simulink library "Game_Development_Library"  (R2024a)
settings: Solver=VariableStepAuto  StartTime=0.0  StopTime=10.0  RelTol=1e-3
libraries: simulink x6
settings Model: Creator=alfa  LastModifiedBy=alfa

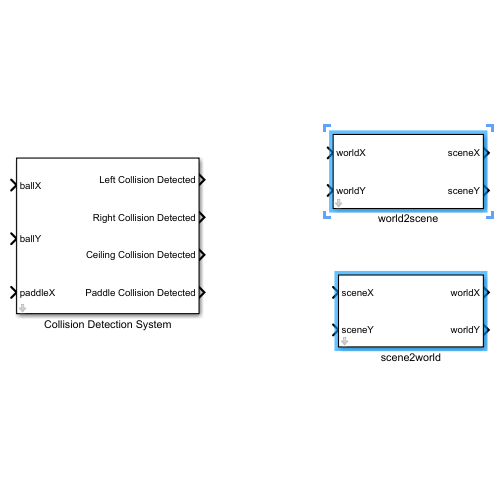
[thumbnail: Simulink's stored preview of the top-level diagram]
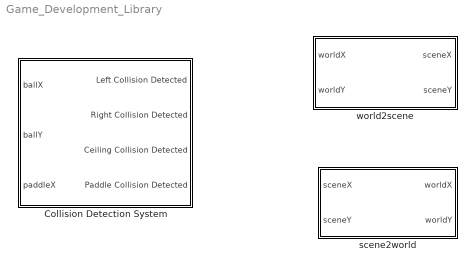
== system Game_Development_Library ==
  Collision Detection System : Subsystem  mask(X- and Y-coordinates of walls and ceilings, width of walls, radius of ball){X_left=-3, X_right=3, w=0.3, Y_ceiling=6, r=0}
      mask prompts: X_left "X-coordinate of left wall"; X_right "X-coordinate of right wall"; w "Width of wall"; Y_ceiling "Y-coordinate of ceiling"; r "Radius of ball"
  scene2world : Subsystem  mask{w=0, h=0}
      mask prompts: w "Width"; h "Height"
  world2scene : Subsystem  mask(world2scene){w=2000, h=250}
      mask prompts: w "Width"; h "Height"

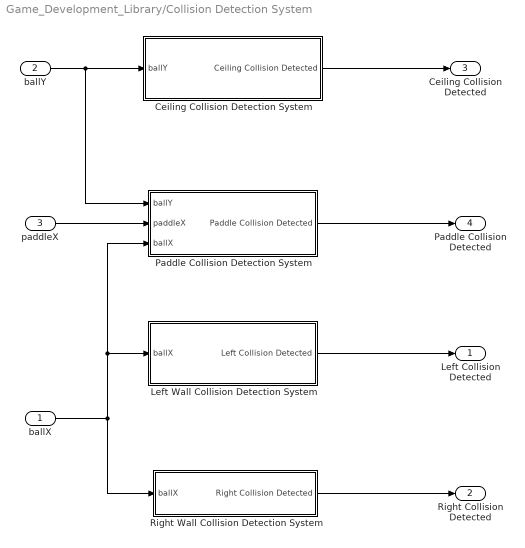
== system Game_Development_Library/Collision Detection System ==
  ballX : Inport
  ballY : Inport  Port=2
  paddleX : Inport  Port=3
  Ceiling Collision Detection System : Subsystem  mask(Y-coordinate used to draw rectangle forming the ceiling, ball radius){Y_ceiling=6, r=0}
      mask prompts: Y_ceiling "Y-coordinate of ceiling"; r "Radius of ball"
  Left Wall Collision Detection System : Subsystem  mask(X-coordinate used to draw rectangle forming the left wall and its' width, ball radius){w=0.3, X_left=-3, r=0}
      mask prompts: w "Width of the wall"; X_left "X-coordinate of left wall"; r "Radius of ball"
  Paddle Collision Detection System : Subsystem  mask{w_paddle=0, h_paddle=0, paddleY=0, r=0}
      mask prompts: w_paddle "Width of paddle"; h_paddle "Height of paddle"; paddleY "Y-coordinate of paddle"; r "Radius of ball"
  Right Wall Collision Detection System : Subsystem  mask(X-coordinate used to draw rectangle forming the right wall, ball radius){X_right=3, r=0}
      mask prompts: X_right "X-coordinate of right wall"; r "Radius of ball"
  Left Collision Detected : Outport
  Right Collision Detected : Outport  Port=2
  Ceiling Collision Detected : Outport  Port=3
  Paddle Collision Detected : Outport  Port=4
  wires:
  Paddle Collision Detection System/1(Paddle Collision Detected) -> Paddle Collision Detected/1
  paddleX/1 -> Paddle Collision Detection System/2(paddleX)
  ballY/1 -> Ceiling Collision Detection System/1(ballY), Paddle Collision Detection System/1(ballY)
  Ceiling Collision Detection System/1(Ceiling Collision Detected) -> Ceiling Collision Detected/1
  Left Wall Collision Detection System/1(Left Collision Detected) -> Left Collision Detected/1
  Right Wall Collision Detection System/1(Right Collision Detected) -> Right Collision Detected/1
  ballX/1 -> Left Wall Collision Detection System/1(ballX), Paddle Collision Detection System/3(ballX), Right Wall Collision Detection System/1(ballX)

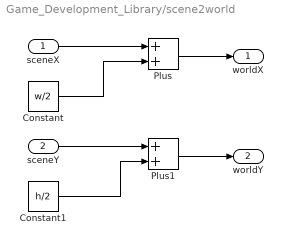
== system Game_Development_Library/scene2world ==
  sceneX : Inport
  "sceneY " : Inport  Port=2
  Constant : Constant  Value=w/2
  Constant1 : Constant  Value=h/2
  Plus : Sum
  Plus1 : Sum
  worldX : Outport
  worldY : Outport  Port=2
  wires:
  Plus1/1 -> worldY/1
  Constant1/1 -> Plus1/2
  Constant/1 -> Plus/2
  Plus/1 -> worldX/1
  sceneX/1 -> Plus/1
  "sceneY "/1 -> Plus1/1

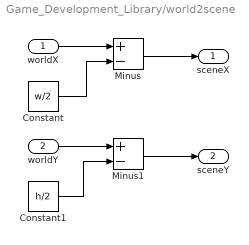
== system Game_Development_Library/world2scene ==
  worldX : Inport
  worldY : Inport  Port=2
  Constant : Constant  Value=w/2
  Constant1 : Constant  Value=h/2
  Minus : Sum  Inputs=+-
  Minus1 : Sum  Inputs=+-
  sceneX : Outport
  sceneY : Outport  Port=2
  wires:
  Minus1/1 -> sceneY/1
  Constant1/1 -> Minus1/2
  worldY/1 -> Minus1/1
  Constant/1 -> Minus/2
  Minus/1 -> sceneX/1
  worldX/1 -> Minus/1

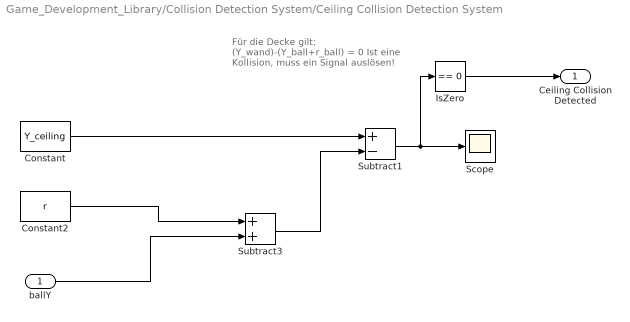
== system Game_Development_Library/Collision Detection System/Ceiling Collision Detection System ==
  note: Für die Decke gilt:
      | (Y_wand)-(Y_ball+r_ball) = 0
      | Ist eine Kollision, muss ein Signal auslösen!
  ballY : Inport
  Constant : Constant  Value=Y_ceiling
  Constant2 : Constant  Value=r
  IsZero : simulink/Logic and Bit Operations/Compare To Zero  relop===  OutDataTypeStr=boolean
      settings: LibrarySourceBlock=|
      | simulink/Quick Insert/Logic and Bit
      | Operations/IsZero
  Scope : Scope
  Subtract1 : Sum  Inputs=+-
  Subtract3 : Sum
  Ceiling Collision Detected : Outport
  wires:
  Constant/1 -> Subtract1/1
  Subtract1/1 -> Scope/1, IsZero/1
  IsZero/1 -> Ceiling Collision Detected/1
  Subtract3/1 -> Subtract1/2
  Constant2/1 -> Subtract3/1
  ballY/1 -> Subtract3/2

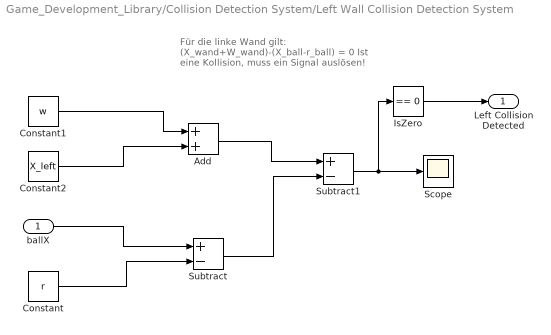
== system Game_Development_Library/Collision Detection System/Left Wall Collision Detection System ==
  note: Für die linke Wand gilt:
      | (X_wand+W_wand)-(X_ball-r_ball) = 0
      | Ist eine Kollision, muss ein Signal auslösen!
  ballX : Inport
  Add : Sum
  Constant : Constant  Value=r
  Constant1 : Constant  Value=w
  Constant2 : Constant  Value=X_left
  IsZero : simulink/Logic and Bit Operations/Compare To Zero  relop===  OutDataTypeStr=boolean
      settings: LibrarySourceBlock=|
      | simulink/Quick Insert/Logic and Bit
      | Operations/IsZero
  Scope : Scope
  Subtract : Sum  Inputs=+-
  Subtract1 : Sum  Inputs=+-
  Left Collision Detected : Outport
  wires:
  Subtract1/1 -> Scope/1, IsZero/1
  ballX/1 -> Subtract/1
  Constant1/1 -> Add/1
  Add/1 -> Subtract1/1
  Constant2/1 -> Add/2
  Subtract/1 -> Subtract1/2
  Constant/1 -> Subtract/2
  IsZero/1 -> Left Collision Detected/1

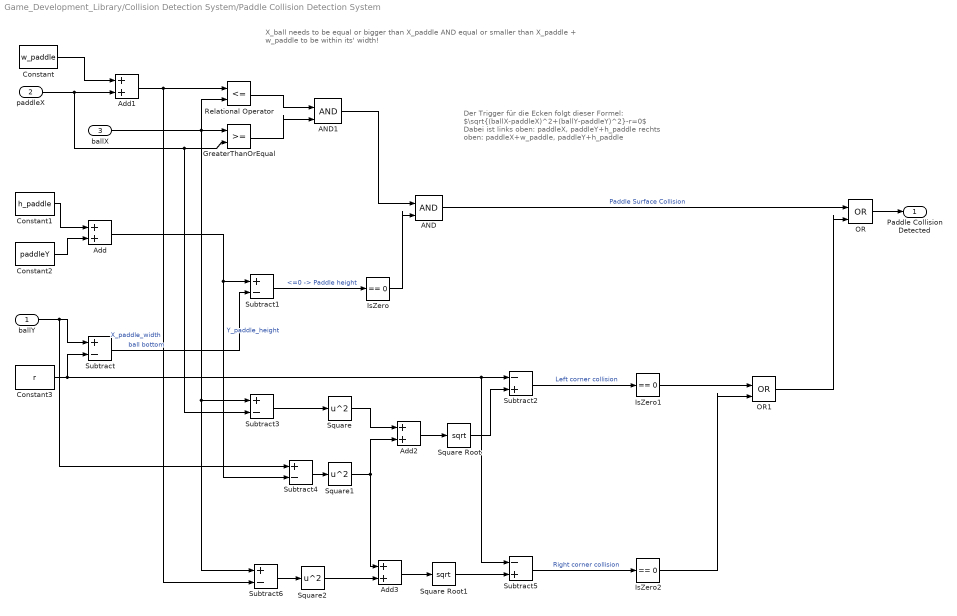
== system Game_Development_Library/Collision Detection System/Paddle Collision Detection System ==
  note: X_ball needs to be equal or bigger than X_paddle AND equal or smaller than X_paddle + w_paddle to be within its' width!
  note: Der Trigger für die Ecken folgt dieser Formel:
      | $\sqrt{(ballX-paddleX)^2+(ballY-paddleY)^2}-r=0$
      |
      | Dabei ist links oben: paddleX, paddleY+h_paddle
      | rechts oben: paddleX+w_paddle, paddleY+h_paddle
  ballY : Inport
  paddleX : Inport  Port=2
  ballX : Inport  Port=3
  AND : Logic  IconShape=distinctive  AllPortsSameDT=off  OutDataTypeStr=boolean
  AND1 : Logic  IconShape=distinctive  AllPortsSameDT=off  OutDataTypeStr=boolean
  Add{,1..3} (4 alike) : Sum
  Constant : Constant  Value=w_paddle
  Constant1 : Constant  Value=h_paddle
  Constant2 : Constant  Value=paddleY
  Constant3 : Constant  Value=r
  GreaterThanOrEqual : RelationalOperator  OutDataTypeStr=boolean  RndMeth=Simplest  InputSameDT=off
  IsZero : simulink/Logic and Bit Operations/Compare To Zero  relop===  OutDataTypeStr=boolean
      settings: LibrarySourceBlock=|
      | simulink/Quick Insert/Logic and Bit
      | Operations/IsZero
  IsZero1 : simulink/Logic and Bit Operations/Compare To Zero  relop===  OutDataTypeStr=boolean
      settings: LibrarySourceBlock=|
      | simulink/Quick Insert/Logic and Bit
      | Operations/IsZero
  IsZero2 : simulink/Logic and Bit Operations/Compare To Zero  relop===  OutDataTypeStr=boolean
      settings: LibrarySourceBlock=|
      | simulink/Quick Insert/Logic and Bit
      | Operations/IsZero
  OR : Logic  Operator=OR  IconShape=distinctive  AllPortsSameDT=off  OutDataTypeStr=boolean
  OR1 : Logic  Operator=OR  IconShape=distinctive  AllPortsSameDT=off  OutDataTypeStr=boolean
  Relational Operator : RelationalOperator  Operator=<=  OutDataTypeStr=boolean  RndMeth=Simplest  InputSameDT=off
  Square : Math  Operator=square
  Square Root : Sqrt
  Square Root1 : Sqrt
  Square1 : Math  Operator=square
  Square2 : Math  Operator=square
  Subtract{,1,3..4,6} (5 alike) : Sum  Inputs=+-
  Subtract2 : Sum  Inputs=-+
  Subtract5 : Sum  Inputs=-+
  Paddle Collision Detected : Outport
  wires:
  Square2/1 -> Add3/2
  Add3/1 -> Square Root1/1
  Subtract5/1 -> IsZero2/1  "Right corner collision"
  Constant3/1 -> Subtract/2, Subtract2/1, Subtract5/1
  IsZero2/1 -> OR1/2
  Subtract6/1 -> Square2/1
  Square Root1/1 -> Subtract5/2
  OR1/1 -> OR/2
  IsZero1/1 -> OR1/1
  Square Root/1 -> Subtract2/2
  Add2/1 -> Square Root/1
  Square1/1 -> Add2/2, Add3/1
  Subtract4/1 -> Square1/1
  Square/1 -> Add2/1
  Subtract3/1 -> Square/1
  Subtract2/1 -> IsZero1/1  "Left corner collision"
  AND/1 -> OR/1  "Paddle Surface Collision"
  OR/1 -> Paddle Collision Detected/1
  AND1/1 -> AND/1
  Relational Operator/1 -> AND1/1
  GreaterThanOrEqual/1 -> AND1/2
  ballX/1 -> GreaterThanOrEqual/1, Subtract3/1, Subtract6/1, Relational Operator/2
  Add1/1 -> Relational Operator/1, Subtract6/2  "X_paddle_width"
  Constant/1 -> Add1/1
  paddleX/1 -> Add1/2, Subtract3/2, GreaterThanOrEqual/2
  IsZero/1 -> AND/2
  Subtract1/1 -> IsZero/1  "<=0 -> Paddle height"
  Subtract/1 -> Subtract1/2  "ball bottom"
  ballY/1 -> Subtract/1, Subtract4/1
  Add/1 -> Subtract4/2, Subtract1/1  "Y_paddle_height"
  Constant2/1 -> Add/2
  Constant1/1 -> Add/1

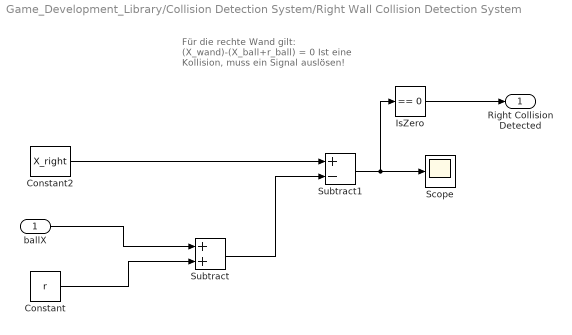
== system Game_Development_Library/Collision Detection System/Right Wall Collision Detection System ==
  note: Für die rechte Wand gilt:
      | (X_wand)-(X_ball+r_ball) = 0
      | Ist eine Kollision, muss ein Signal auslösen!
  ballX : Inport
  Constant : Constant  Value=r
  Constant2 : Constant  Value=X_right
  IsZero : simulink/Logic and Bit Operations/Compare To Zero  relop===  OutDataTypeStr=boolean
      settings: LibrarySourceBlock=|
      | simulink/Quick Insert/Logic and Bit
      | Operations/IsZero
  Scope : Scope
  Subtract : Sum
  Subtract1 : Sum  Inputs=+-
  Right Collision Detected : Outport
  wires:
  Constant/1 -> Subtract/2
  Subtract1/1 -> Scope/1, IsZero/1
  Constant2/1 -> Subtract1/1
  IsZero/1 -> Right Collision Detected/1
  ballX/1 -> Subtract/1
  Subtract/1 -> Subtract1/2
